simulink model "lqr_hover"  (R2021a)
settings: Solver=VariableStepAuto  StartTime=0.0  StopTime=10.0  RelTol=1e-3
values from neighbouring files (symbols this model uses):
  gravity_comp = (9.81 * m)/4    [lqr_script.m]
  K = lqr(A,B, Q,R)    [lqr_script.m]
  setpoint = zeros(n,1)    [lqr_script.m]
libraries: quadcopter_lib x2
settings Model: Creator=ab  LastModifiedBy=ab

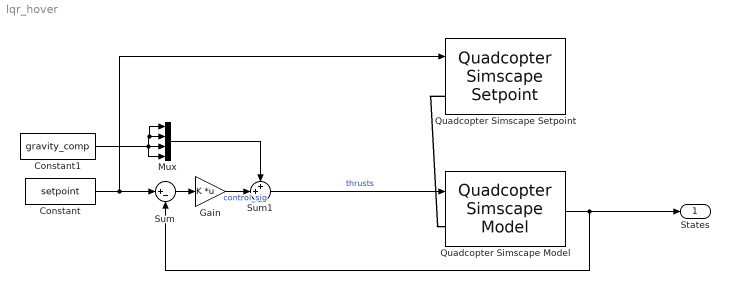
== system lqr_hover ==
  Constant : Constant  Value=setpoint
  Constant1 : Constant  Value=gravity_comp
  Gain : Gain  Gain=K  Multiplication=Matrix(K*u)
  Mux : Mux
  Quadcopter Simscape Model : quadcopter_lib/Quadcopter Simscape Model  box_dim=physical_params.box_dim  box_mass=physical_params.box_mass  arm_dim=physical_params.arm_dim  arm_mass=physical_params.arm_mass  motor_c=physical_params.motor_c  motor_mass=physical_params.motor_mass  throttle_to_thrust=physical_params.throttle_to_thrust  thurst_to_torque=physical_params.thrust_to_torque  g=-9.81
      settings: SourceProductName=Andrew Quadcopter
  Quadcopter Simscape Setpoint : quadcopter_lib/Quadcopter Simscape Setpoint  box_dim=physical_params.box_dim  box_mass=physical_params.box_mass  arm_dim=physical_params.arm_dim  arm_mass=physical_params.arm_mass  motor_c=physical_params.motor_c  motor_mass=physical_params.motor_mass
      settings: SourceProductName=Andrew Quadcopter
  Sum : Sum  Inputs=|+-
  Sum1 : Sum  Inputs=++|
  States : Outport
  wires:
  Quadcopter Simscape Model/1 -> Sum/2, States/1
  Constant/1 -> Quadcopter Simscape Setpoint/1, Sum/1
  Sum1/1 -> Quadcopter Simscape Model/1  "thrusts"
  Constant1/1 -> Mux/4, Mux/1, Mux/2, Mux/3
  Mux/1 -> Sum1/1
  Sum/1 -> Gain/1
  Gain/1 -> Sum1/2  "control_sig"
  connections:
  Quadcopter Simscape Setpoint/LConn1 -- Quadcopter Simscape Model/LConn1
